simulink model "Lab1_2"  (R2024b)
settings: Solver=VariableStepAuto  StartTime=0.0  StopTime=10.0  RelTol=1e-3
settings Model: Creator=Andres Felipe  LastModifiedBy=Andres Felipe

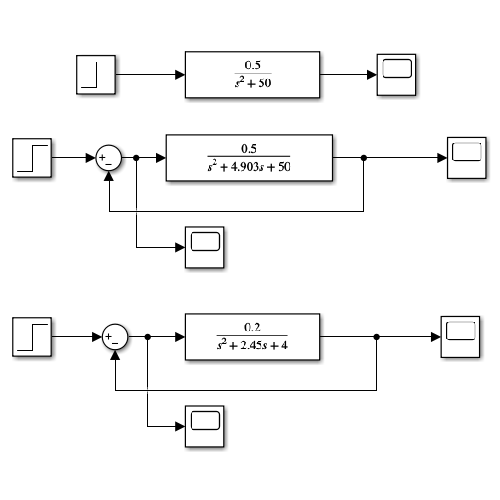
[thumbnail: Simulink's stored preview of the top-level diagram]
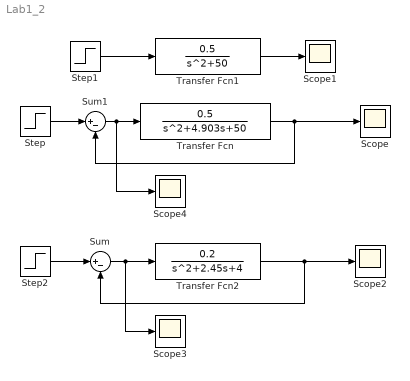
== system Lab1_2 ==
  Scope{,1..4} (5 alike) : Scope
  Step : Step  Time=0  SampleTime=0
  Step1 : Step  Time=0  SampleTime=0
  Step2 : Step  Time=0  SampleTime=0
  Sum : Sum  Inputs=|+-
  Sum1 : Sum  Inputs=|+-
  Transfer Fcn : TransferFcn  Numerator=[0.5]  Denominator=[1 4.903 50]
  Transfer Fcn1 : TransferFcn  Numerator=[0.5]  Denominator=[1 0 50]
  Transfer Fcn2 : TransferFcn  Numerator=[0.2]  Denominator=[1 2.45 4]
  wires:
  Transfer Fcn/1 -> Scope/1, Sum1/2
  Step1/1 -> Transfer Fcn1/1
  Transfer Fcn1/1 -> Scope1/1
  Transfer Fcn2/1 -> Sum/2, Scope2/1
  Sum/1 -> Scope3/1, Transfer Fcn2/1
  Step2/1 -> Sum/1
  Step/1 -> Sum1/1
  Sum1/1 -> Scope4/1, Transfer Fcn/1
